simulink model "MPC_KF"  (R2021b)
settings: Solver=FixedStepDiscrete  StartTime=0.0  StopTime=T_sim  FixedStep=Ts  RelTol=1e-3  EnableMultiTasking=on
values from neighbouring files (symbols this model uses):
  C_states = eye(length(A))    [main.m]
  N5 = 100    [main.m]
  Q5 = Q_d    [main.m]
  R5 = R_d    (= 10000)    [main.m]
  S5 = P_d    [main.m]
  sysd = c2d(sys,T_sampling)    [main.m]
  u_max = deg2rad(15)    [main.m]
  u_min = deg2rad(-15)    [main.m]
  x0 = [deg2rad(0) deg2rad(15) 0 -300]    [main.m]
  x_ref = [0 0 0 0]    [main.m]
undefined symbols (not defined in the file or in its folder): B_noise, D_noise, Discrete, mpc_point_3, NK, RK, Time, Ts, x0K
libraries: simulink x2, ctrlSharedLib x1
settings Model: Creator=Mirko  LastModifiedBy=PaoloA
settings SolverCC: AlgebraicLoopSolver=TrustRegion
settings DataIOCC: LimitDataPoints=on  SaveFormat=Array  SignalLoggingSaveFormat=ModelDataLogs  ReturnWorkspaceOutputs=off
settings OptimizationCC: ExpressionDepthLimit=2147483647  LifeSpan=inf
settings DebuggingCC: UnderspecifiedInitializationDetection=Classic  MergeDetectMultiDrivingBlocksExec=none  FcnCallInpInsideContextMsg=warning  StateNameClashWarn=warning  SFUnexpectedBacktrackingDiag=warning  SFNoUnconditionalDefaultTransitionDiag=warning  SFExecutionAtInitializationDiag=none  SFMachineParentedDataDiag=warning  ArithmeticOperatorsInVariantConditions=warning
settings HardwareCC: ProdBitPerPointer=32  ProdBitPerSizeT=32  ProdBitPerPtrDiffT=32  ProdLargestAtomicFloat=None  ProdIntDivRoundTo=Undefined  ProdEndianess=Unspecified  ProdWordSize=32  ProdHWDeviceType=32-bit Generic
settings ModelReferenceCC: PropagateSignalLabelsOutOfModel=off
settings SFSimCC: SimUseLocalCustomCode=off  CustomCodeUndefinedFunction=UseInterfaceOnly
settings RTWCC: RTWUseLocalCustomCode=off
settings CodeAppCC: StateflowObjectComments=on
settings GRTTargetCC: TargetLangStandard=C89/C90 (ANSI)
settings ConfigComp: CovMetricSettings=dw  CovSaveCumulativeToWorkspaceVar=on  CovSaveSingleToWorkspaceVar=on  CovExternalEMLEnable=off  CovSFcnEnable=off

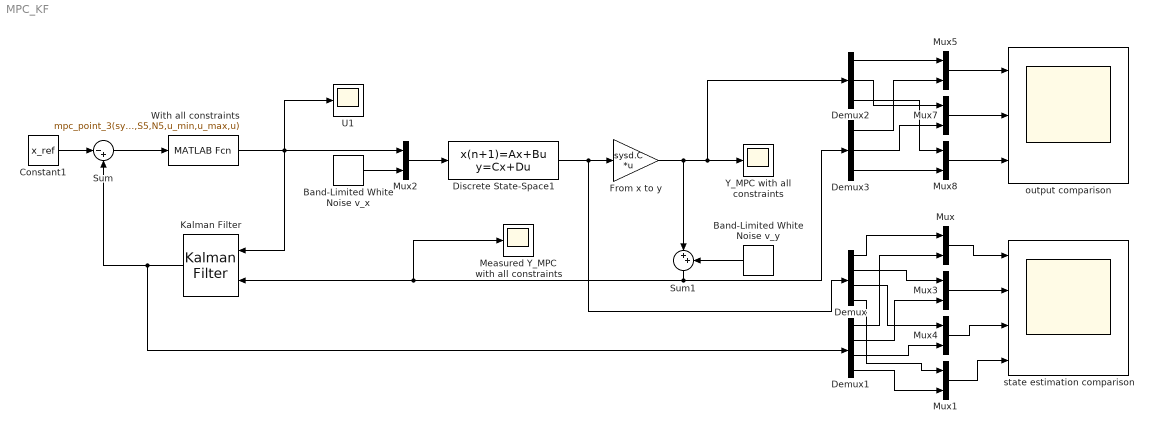
== system MPC_KF ==
  "Band-Limited White Noise v_x " : simulink/Sources/Band-Limited White Noise  Cov=power_vx  Ts=Ts  seed=[23341]
  Band-Limited White Noise v_y : simulink/Sources/Band-Limited White Noise  Cov=power_vy  Ts=Ts  seed=[1258]
  Constant1 : Constant  Value=x_ref
  Demux : Demux
  Demux1 : Demux
  Demux2 : Demux  Outputs=3
  Demux3 : Demux  Outputs=3
  Discrete State-Space1 : DiscreteStateSpace  A=sysd.A  B=B_noise  C=C_states  D=D_noise  InitialCondition=x0  SampleTime=Ts
  From x to y : Gain  Gain=sysd.C  Multiplication=Matrix(K*u)
  Kalman Filter : ctrlSharedLib/Kalman Filter  TimeDomain=Discrete-Time  UseCurrentEstimator=off  ModelSource=Individual A, B, C, D matrices  ModelSourceVariable=ss(0.95,1,1,0,1)  A=sysd.A  B=sysd.B  C=sysd.C  D=sysd.D  NumberOfStates=1  NumberOfInputs=1  NumberOfOutputs=1  InitialEstimateSource=Dialog  X0=x0K  P0=10  UseK=off  UseGH=off  NumberOfProcessNoiseInputs=1  G=1  TimeInvariantG=on  H=0  TimeInvariantH=on  Q=QK  TimeInvariantQ=on  R=RK  TimeInvariantR=on  N=NK  TimeInvariantN=on  AddInputPort=on  AddEnablePort=off  OutputEstimatedY=off  OutputP=off  Ts=Ts
  Measured Y_MPC with all constraints : Scope
  Mux{,1..5,7..8} (8 alike) : Mux  Inputs=2
  Sum : Sum  Inputs=|-+
  Sum1 : Sum  Inputs=|++
  U1 : Scope
  With all constraints : MATLABFcn  MATLABFcn=mpc_point_3(sysd.A,sysd.B,Q5,R5,S5,N5,u_min,u_max,u)  OutputDimensions=1
  Y_MPC with all constraints : Scope
  output comparison : Scope  NumInputPorts=3
  "state estimation comparison " : Scope  NumInputPorts=4
  wires:
  Sum/1 -> With all constraints/1
  From x to y/1 -> Sum1/1, Demux2/1, Y_MPC with all constraints/1
  With all constraints/1 -> Kalman Filter/1, Mux2/1, U1/1
  Constant1/1 -> Sum/1
  "Band-Limited White Noise v_x "/1 -> Mux2/2
  Band-Limited White Noise v_y/1 -> Sum1/2
  Sum1/1 -> Measured Y_MPC with all constraints/1, Kalman Filter/2, Demux3/1
  Kalman Filter/1 -> Demux1/1, Sum/2
  Discrete State-Space1/1 -> From x to y/1, Demux/1
  Demux/1 -> Mux/1
  Demux/2 -> Mux3/1
  Demux/3 -> Mux4/1
  Demux/4 -> Mux1/1
  Demux1/1 -> Mux/2
  Demux1/2 -> Mux3/2
  Demux1/3 -> Mux4/2
  Demux1/4 -> Mux1/2
  Mux/1 -> "state estimation comparison "/1
  Mux3/1 -> "state estimation comparison "/2
  Mux4/1 -> "state estimation comparison "/3
  Mux1/1 -> "state estimation comparison "/4
  Mux2/1 -> Discrete State-Space1/1
  Mux8/1 -> output comparison/3
  Demux2/1 -> Mux5/1
  Mux7/1 -> output comparison/2
  Demux3/2 -> Mux7/2
  Demux2/3 -> Mux8/1
  Demux3/3 -> Mux8/2
  Mux5/1 -> output comparison/1
  Demux3/1 -> Mux5/2
  Demux2/2 -> Mux7/1
